simulink model "encoder2"  (R2012b)
settings: Solver=ode45  StartTime=0.0  StopTime=1  MaxStep=1e-3  RelTol=1e-3
libraries: BLDC x3, Encoder x1
settings Model: Creator=h3now  LastModifiedBy=h3now

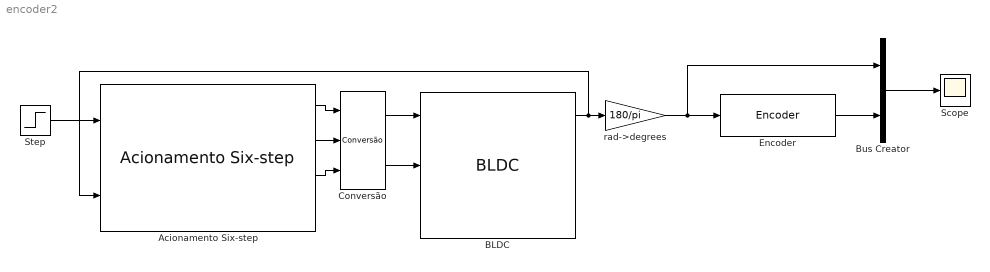
== system encoder2 ==
  Acionamento Six-step : BLDC/Acionamento Six-step  P=8
  BLDC : BLDC/BLDC  J=1.39e-6  R=10.1/2  L=2.04/2000  P=8  Kt=15.7e-3/1.19  Ke=15.7e-3/1.19  Kd=0  F_stick=0  F_slip=0  default_fcem=on  fcem_a=fcem_a  fcem_b=fcem_b  fcem_c=fcem_c
  Bus Creator : BusCreator  Inputs=2
  Conversão : BLDC/Conversão
  Encoder : Encoder/Encoder  Nr=2
  Scope : Scope
      settings: ShowLegends=on
  Step : Step  Time=0.3  Before=3  After=0  SampleTime=0
  rad->degrees : Gain  Gain=180/pi
  wires:
  BLDC/1 -> Acionamento Six-step/2, rad->degrees/1
  Encoder/1 -> Bus Creator/2
  Bus Creator/1 -> Scope/1
  rad->degrees/1 -> Bus Creator/1, Encoder/1
  Conversão/2 -> BLDC/2
  Conversão/1 -> BLDC/1
  Acionamento Six-step/2 -> Conversão/2
  Acionamento Six-step/3 -> Conversão/3
  Acionamento Six-step/1 -> Conversão/1
  Step/1 -> Acionamento Six-step/1
